simulink model "motor_simx"  (R2020b)
settings: Solver=ode45  StartTime=0.0  StopTime=34  RelTol=1e-3  EnableMultiTasking=on
PreLoadFcn:
  | MotorParam
InitFcn:
  | MotorParam
values from neighbouring files (symbols this model uses):
  B = (Km*INL)/w    (= 4.14319136746e-07)    [MotorParam.m]
  J = Rotor_inertia    (= 2.23668e-07)    [MotorParam.m]
  Kb = (Speed_constant)/(.10472)    (= 0.0177826336223)    [MotorParam.m]
  Km = Torque_constant*1E-3    (= 0.0178)    [MotorParam.m]
  L = Terminal_inductance*1E-3    (= 0.000411)    [MotorParam.m]
  R = Terminal_resistance    (= 5.82)    [MotorParam.m]
libraries: pid_lib x4, simulink x1
settings Model: Creator=Leo  LastModifiedBy=Jeff
settings DataIOCC: LimitDataPoints=on  SaveFormat=Array  SignalLoggingSaveFormat=ModelDataLogs  ReturnWorkspaceOutputs=off
settings OptimizationCC: ExpressionDepthLimit=2147483647  InitFltsAndDblsToZero=on  LifeSpan=inf
settings DebuggingCC: UnderspecifiedInitializationDetection=Classic  MergeDetectMultiDrivingBlocksExec=none  SolverPrmCheckMsg=warning  FcnCallInpInsideContextMsg=warning  StateNameClashWarn=warning  SFUnexpectedBacktrackingDiag=warning  SFNoUnconditionalDefaultTransitionDiag=warning  SFExecutionAtInitializationDiag=none  ArithmeticOperatorsInVariantConditions=warning
settings HardwareCC: ProdBitPerPointer=32  ProdBitPerSizeT=32  ProdBitPerPtrDiffT=32  ProdLargestAtomicFloat=None  ProdIntDivRoundTo=Undefined  ProdEndianess=Unspecified  ProdWordSize=32  ProdHWDeviceType=32-bit Generic
settings ModelReferenceCC: PropagateSignalLabelsOutOfModel=off
settings SFSimCC: SimUseLocalCustomCode=off  CustomCodeUndefinedFunction=UseInterfaceOnly
settings RTWCC: RTWUseLocalCustomCode=off
settings CodeAppCC: StateflowObjectComments=on
settings GRTTargetCC: TargetLangStandard=C89/C90 (ANSI)  CombineOutputUpdateFcns=off  GRTInterface=on
settings ConfigComp: CovMetricSettings=dw  CovSaveCumulativeToWorkspaceVar=on  CovSaveSingleToWorkspaceVar=on  CovExternalEMLEnable=off  CovSFcnEnable=off

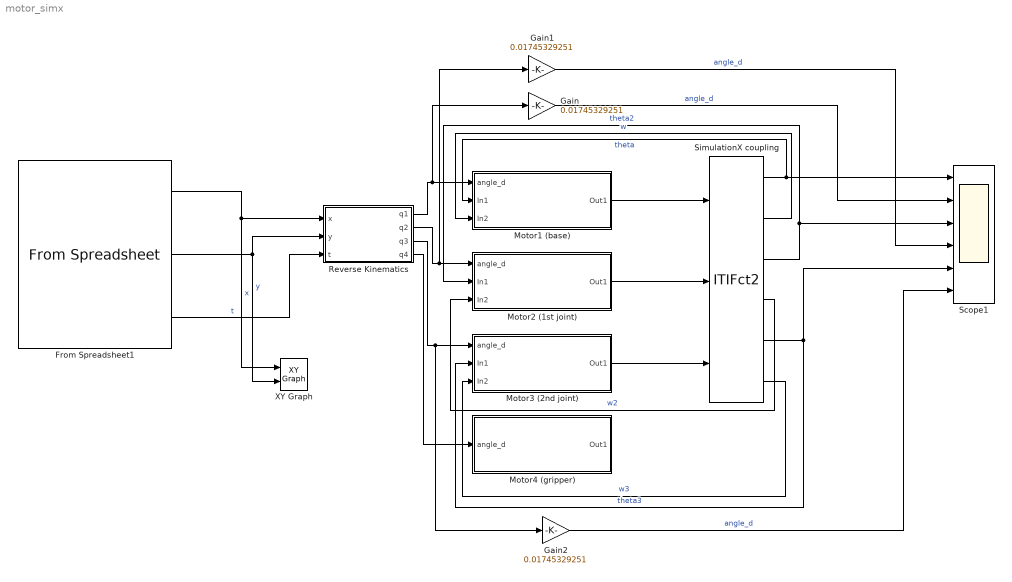
== system motor_simx ==
  From Spreadsheet1 : FromSpreadsheet  FileName=Motor_pos.xlsx
  Gain : Gain  Gain=0.01745329251
  Gain1 : Gain  Gain=0.01745329251
  Gain2 : Gain  Gain=0.01745329251
  Motor1 (base) : Subsystem
  Motor2 (1st joint) : Subsystem
  Motor3 (2nd joint) : Subsystem
  Motor4 (gripper) : Subsystem
  Reverse Kinematics : MATLAB Function  TreatAsAtomicUnit=on
  Scope1 : Scope  NumInputPorts=6
  SimulationX coupling : S-Function  FunctionName=ITIFct2  Parameters=ip, port, ts, nIn, nOut  SFunctionDeploymentMode=off  EnableBusSupport=off  mask{ip="localhost", port=4097, ts=0.001, nIn=3, nOut=6}
      mask prompts: ip "Address: ip"; port "Port Number: port [-]"; ts "Communication Step Size: ts [s]"; nIn "Input Vector Dimension (to SimulationX): nIn [-]"; nOut "Output Vector Dimension (from SimulationX): nOut [-]"
      mask help: Coupling Element
  XY Graph : simulink/Sinks/XY Graph  xmin=-15  xmax=15  ymin=-5  ymax=50  st=0.001
  wires:
  From Spreadsheet1/1 -> XY Graph/1, Reverse Kinematics/1(x)  "x"
  Motor1 (base)/1(Out1) -> SimulationX coupling/1
  From Spreadsheet1/2 -> XY Graph/2, Reverse Kinematics/2(y)  "y"
  Reverse Kinematics/1(q1) -> Gain/1, Motor1 (base)/1(angle_d)
  Reverse Kinematics/4(q4) -> Motor4 (gripper)/1(angle_d)
  From Spreadsheet1/3 -> Reverse Kinematics/3(t)  "t"
  SimulationX coupling/1 -> Motor1 (base)/2(In1), Scope1/1  "theta"
  SimulationX coupling/2 -> Motor1 (base)/3(In2)  "w"
  Reverse Kinematics/2(q2) -> Gain1/1, Motor2 (1st joint)/1(angle_d)
  Reverse Kinematics/3(q3) -> Gain2/1, Motor3 (2nd joint)/1(angle_d)
  SimulationX coupling/3 -> Scope1/3, Motor2 (1st joint)/2(In1)  "theta2"
  SimulationX coupling/4 -> Motor2 (1st joint)/3(In2)  "w2"
  SimulationX coupling/5 -> Motor3 (2nd joint)/2(In1), Scope1/5  "theta3"
  SimulationX coupling/6 -> Motor3 (2nd joint)/3(In2)  "w3"
  Motor2 (1st joint)/1(Out1) -> SimulationX coupling/2
  Motor3 (2nd joint)/1(Out1) -> SimulationX coupling/3
  Gain/1 -> Scope1/2  "angle_d"
  Gain1/1 -> Scope1/4  "angle_d"
  Gain2/1 -> Scope1/6  "angle_d"

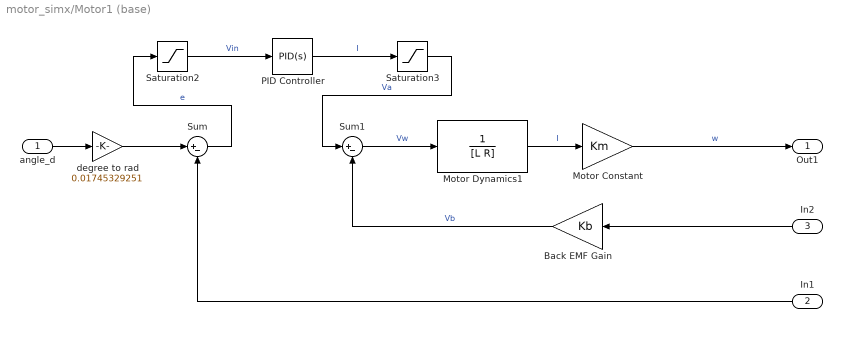
== system motor_simx/Motor1 (base) ==
  angle_d : Inport
  In1 : Inport  Port=2
  In2 : Inport  Port=3
  Back EMF Gain : Gain  Gain=Kb
  Motor Constant : Gain  Gain=Km
  Motor Dynamics1 : TransferFcn  Denominator=[L R]
  PID Controller : pid_lib/PID Controller  Controller=PID  Form=Parallel  TimeDomain=Continuous-time  UseExternalTs=off  SampleTime=-1  IntegratorMethod=Forward Euler  FilterMethod=Forward Euler  ControllerParametersSource=internal  P=100  I=0  D=100  UseFilter=on  N=100  TunerSelectOption=Transfer Function Based (PID Tuner App)  InitialConditionSource=internal  InitialConditionForIntegrator=0  InitialConditionForFilter=0  DifferentiatorICPrevScaledInput=0  ExternalReset=none  TrackingMode=off  Kt=1  LimitOutput=off  SatLimitsSource=internal  UpperSaturationLimit=inf  LowerSaturationLimit=-inf  LinearizeAsGain=on  AntiWindupMode=none  Kb=1  POutMin=[]  POutMax=[]  IOutMin=[]  IOutMax=[]  DOutMin=[]  DOutMax=[]  NOutMin=[]  NOutMax=[]  SumOutMin=[]  SumOutMax=[]  SaturationOutMin=[]  SaturationOutMax=[]  PParamMin=[]  PParamMax=[]  IParamMin=[]  IParamMax=[]  DParamMin=[]  DParamMax=[]  NParamMin=[]  NParamMax=[]  KbParamMin=[]  KbParamMax=[]  KtParamMin=[]  KtParamMax=[]  KbOutMin=[]  KbOutMax=[]  KtOutMin=[]  KtOutMax=[]  IntegratorOutMin=[]  IntegratorOutMax=[]  FilterOutMin=[]  FilterOutMax=[]  SumI1OutMin=[]  SumI1OutMax=[]  SumI2OutMin=[]  SumI2OutMax=[]  SumI3OutMin=[]  SumI3OutMax=[]  SumI4OutMin=[]  SumI4OutMax=[]  SumDOutMin=[]  SumDOutMax=[]  DifferentiatorOutMin=[]  DifferentiatorOutMax=[]  FilterDiffOutCoefMin=[]  FilterDiffOutCoefMax=[]  ReciprocalOutMin=[]  ReciprocalOutMax=[]  SumDenOutMin=[]  SumDenOutMax=[]  SumNumOutMin=[]  SumNumOutMax=[]  DivideOutMin=[]  DivideOutMax=[]  UdiffTsProdOutMin=[]  UdiffTsProdOutMax=[]  NTsProdOutMin=[]  NTsProdOutMax=[]  UintegralTsProdOutMin=[]  UintegralTsProdOutMax=[]  UngainTsProdOutMin=[]  UngainTsProdOutMax=[]  IntegratorContinuousStateAttributes=''  IntegratorStateMustResolveToSignalObject=off  IntegratorRTWStateStorageClass=Auto  FilterContinuousStateAttributes=''  FilterStateMustResolveToSignalObject=off  FilterRTWStateStorageClass=Auto  ParallelPVariant=InternalParameters  IdealPVariant=Disabled  IVariant=InternalParameters  DVariant=InternalParameters  IntegratorVariant=Continuous  SatVariant=Disabled  AWVariant=Passthrough  PCopyVariant=Disabled  TRVariant=Disabled  FdbkBlocksVariant=Forward  IdealPFdbkVariant=Disabled  SatFdbkVariant=Disabled  DerivativeFilterVariant=ContFilter  NVariant=InternalParameters  NCopyVariant=Disabled  FilterICVariant=InternalICsFilter  IntegratorICVariant=InternalICs  ExternalResetVariant=Disabled  TRSumVariant=Passthrough  SumFdbkVariant=Disabled  SumVariant=Sum_PID  TsampFilterVariant=InternalTs  TsampNgainVariant=Passthrough  TsampIntegralVariant=Passthrough  ExternalSaturationOutDataTypeStr=Inherit: Same as second input
  Saturation2 : Saturate  UpperLimit=5  LowerLimit=-5
  Saturation3 : Saturate  UpperLimit=18  LowerLimit=-18
  Sum : Sum  Inputs=|+-
  Sum1 : Sum  Inputs=|+-
  degree to rad : Gain  Gain=0.01745329251
  Out1 : Outport
  wires:
  angle_d/1 -> degree to rad/1
  Sum/1 -> Saturation2/1  "e"
  Motor Constant/1 -> Out1/1  "w"
  Back EMF Gain/1 -> Sum1/2  "Vb"
  Motor Dynamics1/1 -> Motor Constant/1  "I"
  Sum1/1 -> Motor Dynamics1/1  "Vw"
  In1/1 -> Sum/2
  In2/1 -> Back EMF Gain/1
  PID Controller/1 -> Saturation3/1  "I"
  Saturation2/1 -> PID Controller/1  "Vin"
  Saturation3/1 -> Sum1/1  "Va"
  degree to rad/1 -> Sum/1

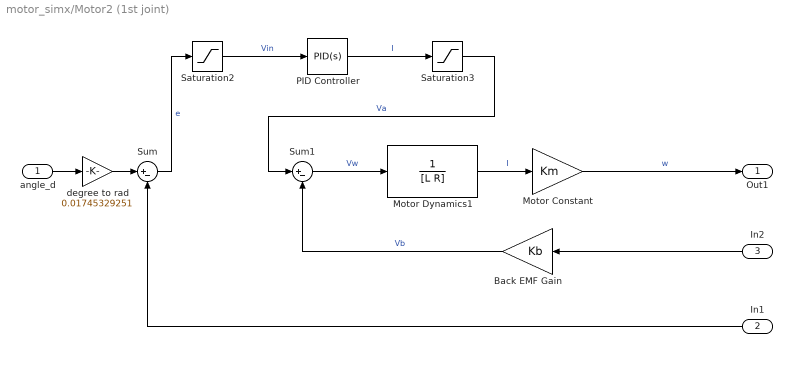
== system motor_simx/Motor2 (1st joint) ==
  angle_d : Inport
  In1 : Inport  Port=2
  In2 : Inport  Port=3
  Back EMF Gain : Gain  Gain=Kb
  Motor Constant : Gain  Gain=Km
  Motor Dynamics1 : TransferFcn  Denominator=[L R]
  PID Controller : pid_lib/PID Controller  Controller=PID  Form=Parallel  TimeDomain=Continuous-time  UseExternalTs=off  SampleTime=-1  IntegratorMethod=Forward Euler  FilterMethod=Forward Euler  ControllerParametersSource=internal  P=100  I=0  D=100  UseFilter=on  N=100  TunerSelectOption=Transfer Function Based (PID Tuner App)  InitialConditionSource=internal  InitialConditionForIntegrator=0  InitialConditionForFilter=0  DifferentiatorICPrevScaledInput=0  ExternalReset=none  TrackingMode=off  Kt=1  LimitOutput=off  SatLimitsSource=internal  UpperSaturationLimit=inf  LowerSaturationLimit=-inf  LinearizeAsGain=on  AntiWindupMode=none  Kb=1  POutMin=[]  POutMax=[]  IOutMin=[]  IOutMax=[]  DOutMin=[]  DOutMax=[]  NOutMin=[]  NOutMax=[]  SumOutMin=[]  SumOutMax=[]  SaturationOutMin=[]  SaturationOutMax=[]  PParamMin=[]  PParamMax=[]  IParamMin=[]  IParamMax=[]  DParamMin=[]  DParamMax=[]  NParamMin=[]  NParamMax=[]  KbParamMin=[]  KbParamMax=[]  KtParamMin=[]  KtParamMax=[]  KbOutMin=[]  KbOutMax=[]  KtOutMin=[]  KtOutMax=[]  IntegratorOutMin=[]  IntegratorOutMax=[]  FilterOutMin=[]  FilterOutMax=[]  SumI1OutMin=[]  SumI1OutMax=[]  SumI2OutMin=[]  SumI2OutMax=[]  SumI3OutMin=[]  SumI3OutMax=[]  SumI4OutMin=[]  SumI4OutMax=[]  SumDOutMin=[]  SumDOutMax=[]  DifferentiatorOutMin=[]  DifferentiatorOutMax=[]  FilterDiffOutCoefMin=[]  FilterDiffOutCoefMax=[]  ReciprocalOutMin=[]  ReciprocalOutMax=[]  SumDenOutMin=[]  SumDenOutMax=[]  SumNumOutMin=[]  SumNumOutMax=[]  DivideOutMin=[]  DivideOutMax=[]  UdiffTsProdOutMin=[]  UdiffTsProdOutMax=[]  NTsProdOutMin=[]  NTsProdOutMax=[]  UintegralTsProdOutMin=[]  UintegralTsProdOutMax=[]  UngainTsProdOutMin=[]  UngainTsProdOutMax=[]  IntegratorContinuousStateAttributes=''  IntegratorStateMustResolveToSignalObject=off  IntegratorRTWStateStorageClass=Auto  FilterContinuousStateAttributes=''  FilterStateMustResolveToSignalObject=off  FilterRTWStateStorageClass=Auto  ParallelPVariant=InternalParameters  IdealPVariant=Disabled  IVariant=InternalParameters  DVariant=InternalParameters  IntegratorVariant=Continuous  SatVariant=Disabled  AWVariant=Passthrough  PCopyVariant=Disabled  TRVariant=Disabled  FdbkBlocksVariant=Forward  IdealPFdbkVariant=Disabled  SatFdbkVariant=Disabled  DerivativeFilterVariant=ContFilter  NVariant=InternalParameters  NCopyVariant=Disabled  FilterICVariant=InternalICsFilter  IntegratorICVariant=InternalICs  ExternalResetVariant=Disabled  TRSumVariant=Passthrough  SumFdbkVariant=Disabled  SumVariant=Sum_PID  TsampFilterVariant=InternalTs  TsampNgainVariant=Passthrough  TsampIntegralVariant=Passthrough  ExternalSaturationOutDataTypeStr=Inherit: Same as second input
  Saturation2 : Saturate  UpperLimit=5  LowerLimit=-5
  Saturation3 : Saturate  UpperLimit=18  LowerLimit=-18
  Sum : Sum  Inputs=|+-
  Sum1 : Sum  Inputs=|+-
  degree to rad : Gain  Gain=0.01745329251
  Out1 : Outport
  wires:
  Back EMF Gain/1 -> Sum1/2  "Vb"
  Sum/1 -> Saturation2/1  "e"
  In1/1 -> Sum/2
  Motor Constant/1 -> Out1/1  "w"
  Motor Dynamics1/1 -> Motor Constant/1  "I"
  In2/1 -> Back EMF Gain/1
  angle_d/1 -> degree to rad/1
  Sum1/1 -> Motor Dynamics1/1  "Vw"
  PID Controller/1 -> Saturation3/1  "I"
  Saturation2/1 -> PID Controller/1  "Vin"
  Saturation3/1 -> Sum1/1  "Va"
  degree to rad/1 -> Sum/1

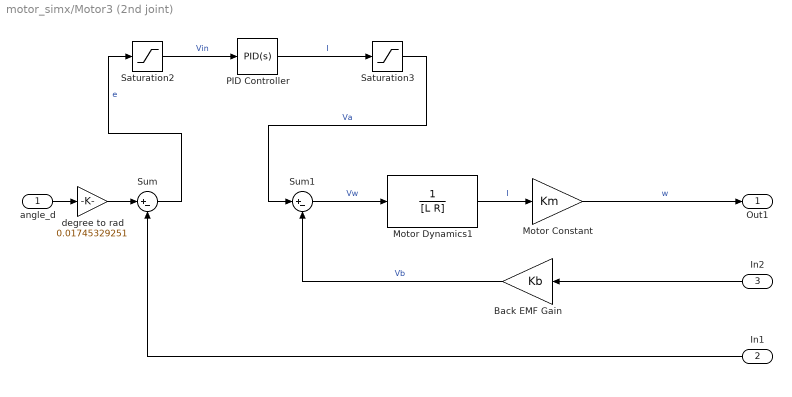
== system motor_simx/Motor3 (2nd joint) ==
  angle_d : Inport
  In1 : Inport  Port=2
  In2 : Inport  Port=3
  Back EMF Gain : Gain  Gain=Kb
  Motor Constant : Gain  Gain=Km
  Motor Dynamics1 : TransferFcn  Denominator=[L R]
  PID Controller : pid_lib/PID Controller  Controller=PID  Form=Parallel  TimeDomain=Continuous-time  UseExternalTs=off  SampleTime=-1  IntegratorMethod=Forward Euler  FilterMethod=Forward Euler  ControllerParametersSource=internal  P=1  I=0  D=5  UseFilter=on  N=100  TunerSelectOption=Transfer Function Based (PID Tuner App)  InitialConditionSource=internal  InitialConditionForIntegrator=0  InitialConditionForFilter=0  DifferentiatorICPrevScaledInput=0  ExternalReset=none  TrackingMode=off  Kt=1  LimitOutput=off  SatLimitsSource=internal  UpperSaturationLimit=inf  LowerSaturationLimit=-inf  LinearizeAsGain=on  AntiWindupMode=none  Kb=1  POutMin=[]  POutMax=[]  IOutMin=[]  IOutMax=[]  DOutMin=[]  DOutMax=[]  NOutMin=[]  NOutMax=[]  SumOutMin=[]  SumOutMax=[]  SaturationOutMin=[]  SaturationOutMax=[]  PParamMin=[]  PParamMax=[]  IParamMin=[]  IParamMax=[]  DParamMin=[]  DParamMax=[]  NParamMin=[]  NParamMax=[]  KbParamMin=[]  KbParamMax=[]  KtParamMin=[]  KtParamMax=[]  KbOutMin=[]  KbOutMax=[]  KtOutMin=[]  KtOutMax=[]  IntegratorOutMin=[]  IntegratorOutMax=[]  FilterOutMin=[]  FilterOutMax=[]  SumI1OutMin=[]  SumI1OutMax=[]  SumI2OutMin=[]  SumI2OutMax=[]  SumI3OutMin=[]  SumI3OutMax=[]  SumI4OutMin=[]  SumI4OutMax=[]  SumDOutMin=[]  SumDOutMax=[]  DifferentiatorOutMin=[]  DifferentiatorOutMax=[]  FilterDiffOutCoefMin=[]  FilterDiffOutCoefMax=[]  ReciprocalOutMin=[]  ReciprocalOutMax=[]  SumDenOutMin=[]  SumDenOutMax=[]  SumNumOutMin=[]  SumNumOutMax=[]  DivideOutMin=[]  DivideOutMax=[]  UdiffTsProdOutMin=[]  UdiffTsProdOutMax=[]  NTsProdOutMin=[]  NTsProdOutMax=[]  UintegralTsProdOutMin=[]  UintegralTsProdOutMax=[]  UngainTsProdOutMin=[]  UngainTsProdOutMax=[]  IntegratorContinuousStateAttributes=''  IntegratorStateMustResolveToSignalObject=off  IntegratorRTWStateStorageClass=Auto  FilterContinuousStateAttributes=''  FilterStateMustResolveToSignalObject=off  FilterRTWStateStorageClass=Auto  ParallelPVariant=InternalParameters  IdealPVariant=Disabled  IVariant=InternalParameters  DVariant=InternalParameters  IntegratorVariant=Continuous  SatVariant=Disabled  AWVariant=Passthrough  PCopyVariant=Disabled  TRVariant=Disabled  FdbkBlocksVariant=Forward  IdealPFdbkVariant=Disabled  SatFdbkVariant=Disabled  DerivativeFilterVariant=ContFilter  NVariant=InternalParameters  NCopyVariant=Disabled  FilterICVariant=InternalICsFilter  IntegratorICVariant=InternalICs  ExternalResetVariant=Disabled  TRSumVariant=Passthrough  SumFdbkVariant=Disabled  SumVariant=Sum_PID  TsampFilterVariant=InternalTs  TsampNgainVariant=Passthrough  TsampIntegralVariant=Passthrough  ExternalSaturationOutDataTypeStr=Inherit: Same as second input
  Saturation2 : Saturate  UpperLimit=5  LowerLimit=-5
  Saturation3 : Saturate  UpperLimit=18  LowerLimit=-18
  Sum : Sum  Inputs=|+-
  Sum1 : Sum  Inputs=|+-
  degree to rad : Gain  Gain=0.01745329251
  Out1 : Outport
  wires:
  Back EMF Gain/1 -> Sum1/2  "Vb"
  Sum/1 -> Saturation2/1  "e"
  In1/1 -> Sum/2
  Motor Constant/1 -> Out1/1  "w"
  Motor Dynamics1/1 -> Motor Constant/1  "I"
  In2/1 -> Back EMF Gain/1
  angle_d/1 -> degree to rad/1
  Sum1/1 -> Motor Dynamics1/1  "Vw"
  PID Controller/1 -> Saturation3/1  "I"
  Saturation2/1 -> PID Controller/1  "Vin"
  Saturation3/1 -> Sum1/1  "Va"
  degree to rad/1 -> Sum/1

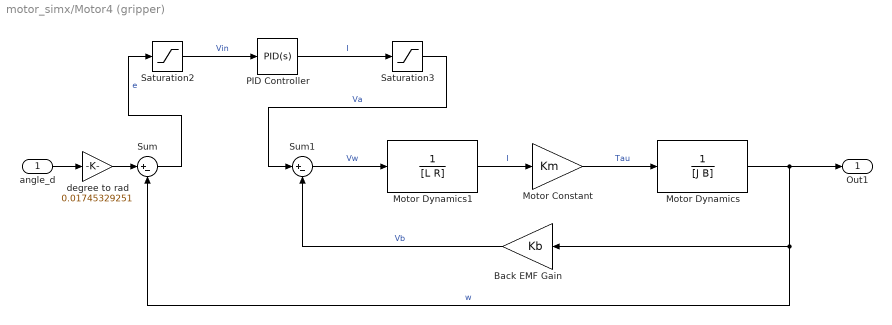
== system motor_simx/Motor4 (gripper) ==
  angle_d : Inport
  Back EMF Gain : Gain  Gain=Kb
  Motor Constant : Gain  Gain=Km
  Motor Dynamics : TransferFcn  Denominator=[J B]
  Motor Dynamics1 : TransferFcn  Denominator=[L R]
  PID Controller : pid_lib/PID Controller  Controller=PID  Form=Parallel  TimeDomain=Continuous-time  UseExternalTs=off  SampleTime=-1  IntegratorMethod=Forward Euler  FilterMethod=Forward Euler  ControllerParametersSource=internal  P=20  I=0  D=15  UseFilter=on  N=100  TunerSelectOption=Transfer Function Based (PID Tuner App)  InitialConditionSource=internal  InitialConditionForIntegrator=0  InitialConditionForFilter=0  DifferentiatorICPrevScaledInput=0  ExternalReset=none  TrackingMode=off  Kt=1  LimitOutput=off  SatLimitsSource=internal  UpperSaturationLimit=inf  LowerSaturationLimit=-inf  LinearizeAsGain=on  AntiWindupMode=none  Kb=1  POutMin=[]  POutMax=[]  IOutMin=[]  IOutMax=[]  DOutMin=[]  DOutMax=[]  NOutMin=[]  NOutMax=[]  SumOutMin=[]  SumOutMax=[]  SaturationOutMin=[]  SaturationOutMax=[]  PParamMin=[]  PParamMax=[]  IParamMin=[]  IParamMax=[]  DParamMin=[]  DParamMax=[]  NParamMin=[]  NParamMax=[]  KbParamMin=[]  KbParamMax=[]  KtParamMin=[]  KtParamMax=[]  KbOutMin=[]  KbOutMax=[]  KtOutMin=[]  KtOutMax=[]  IntegratorOutMin=[]  IntegratorOutMax=[]  FilterOutMin=[]  FilterOutMax=[]  SumI1OutMin=[]  SumI1OutMax=[]  SumI2OutMin=[]  SumI2OutMax=[]  SumI3OutMin=[]  SumI3OutMax=[]  SumI4OutMin=[]  SumI4OutMax=[]  SumDOutMin=[]  SumDOutMax=[]  DifferentiatorOutMin=[]  DifferentiatorOutMax=[]  FilterDiffOutCoefMin=[]  FilterDiffOutCoefMax=[]  ReciprocalOutMin=[]  ReciprocalOutMax=[]  SumDenOutMin=[]  SumDenOutMax=[]  SumNumOutMin=[]  SumNumOutMax=[]  DivideOutMin=[]  DivideOutMax=[]  UdiffTsProdOutMin=[]  UdiffTsProdOutMax=[]  NTsProdOutMin=[]  NTsProdOutMax=[]  UintegralTsProdOutMin=[]  UintegralTsProdOutMax=[]  UngainTsProdOutMin=[]  UngainTsProdOutMax=[]  IntegratorContinuousStateAttributes=''  IntegratorStateMustResolveToSignalObject=off  IntegratorRTWStateStorageClass=Auto  FilterContinuousStateAttributes=''  FilterStateMustResolveToSignalObject=off  FilterRTWStateStorageClass=Auto  ParallelPVariant=InternalParameters  IdealPVariant=Disabled  IVariant=InternalParameters  DVariant=InternalParameters  IntegratorVariant=Continuous  SatVariant=Disabled  AWVariant=Passthrough  PCopyVariant=Disabled  TRVariant=Disabled  FdbkBlocksVariant=Forward  IdealPFdbkVariant=Disabled  SatFdbkVariant=Disabled  DerivativeFilterVariant=ContFilter  NVariant=InternalParameters  NCopyVariant=Disabled  FilterICVariant=InternalICsFilter  IntegratorICVariant=InternalICs  ExternalResetVariant=Disabled  TRSumVariant=Passthrough  SumFdbkVariant=Disabled  SumVariant=Sum_PID  TsampFilterVariant=InternalTs  TsampNgainVariant=Passthrough  TsampIntegralVariant=Passthrough  ExternalSaturationOutDataTypeStr=Inherit: Same as second input
  Saturation2 : Saturate  UpperLimit=5  LowerLimit=-5
  Saturation3 : Saturate  UpperLimit=18  LowerLimit=-18
  Sum : Sum  Inputs=|+-
  Sum1 : Sum  Inputs=|+-
  degree to rad : Gain  Gain=0.01745329251
  Out1 : Outport
  wires:
  angle_d/1 -> degree to rad/1
  Motor Dynamics/1 -> Out1/1, Sum/2, Back EMF Gain/1  "w"
  Motor Constant/1 -> Motor Dynamics/1  "Tau"
  Back EMF Gain/1 -> Sum1/2  "Vb"
  Motor Dynamics1/1 -> Motor Constant/1  "I"
  Sum1/1 -> Motor Dynamics1/1  "Vw"
  PID Controller/1 -> Saturation3/1  "I"
  Saturation2/1 -> PID Controller/1  "Vin"
  Sum/1 -> Saturation2/1  "e"
  Saturation3/1 -> Sum1/1  "Va"
  degree to rad/1 -> Sum/1

== matlab function motor_simx/Reverse Kinematics ==
  data: x input; y input; t input; q1 output; q2 output; q3 output; q4 output
    function [q1, q2, q3, q4]= fcn(x,y,t)
    a1 = 20;
    a2 = 30;
    
    q2 = acosd((x^2+y^2-a1^2-a2^2)/(2*a1*a2));
    q1 = atand(y/x)-atand(a2*sind(q2)/(a1+a2*cosd(q2)));
    q4 = 0;
    if q1<0 
        q1 = 180+q1;
    end
    q3 = 180-q1-q2;
    if q3<0
        q3 = 90;
    end
    
    if x==-10 && y==40 && t>=6 && t<=8
        % close gripper
        q4 = 180;
    end
    if x==-10 && y==30 && t>=10 && t<=12
        % open gripper
        q4 = 0;
    end
    
    if x==0 && y==40 && t>=16 && t<=18
        % close gripper
        q4 = 180;
    end
    if x==0 && y==30 && t>=20 && t<=22
        % open gripper
        q4 = 0;
    end
    
    if x==10 && y==40 && t>=26 && t<=28
        % close gripper
        q4 = 180;
    end
    if x==10 && y==30 && t>=30 && t<=32
        % open gripper
        q4 = 0;
    end
